simulink model "ASM_Losses"  (R2014a)
settings: Solver=ode23t  StartTime=0.0  StopTime=1/input.fs*3  MaxStep=1e-3  MinStep=1e-12  RelTol=1e-3
undefined symbols (not defined in the file or in its folder): input, motor, pwm
libraries: fl_lib x24, nesl_utility x20, elec_lib x2, simulink x2, powerlib_meascontrol x1
settings Model: Creator=sizuest  LastModifiedBy=simon
settings SolverCC: MaxConsecutiveMinStep=10
settings DataIOCC: SignalLoggingSaveFormat=ModelDataLogs
settings DebuggingCC: UnderspecifiedInitializationDetection=Classic  MaxConsecutiveZCsMsg=none  IgnoredZcDiagnostic=none  MultiTaskDSMMsg=warning  MultiTaskCondExecSysMsg=none  ParameterPrecisionLossMsg=none
settings RTWCC: IncludeERTFirstTime=on

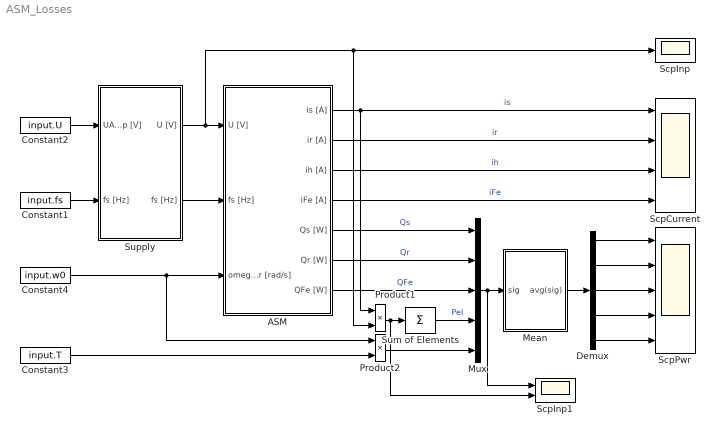
== system ASM_Losses ==
  ASM : Subsystem
  Constant1 : Constant  Value=input.fs
  Constant2 : Constant  Value=input.U
  Constant3 : Constant  Value=input.T
  Constant4 : Constant  Value=input.w0
  Demux : Demux  Outputs=5
  Mean : Subsystem
  Mux : Mux  Inputs=5
  Product1 : Product
  Product2 : Product
  ScpCurrent : Scope  NumInputPorts=4
      settings: ShowLegends=on  TimeRange=0.00432192  YMin=-100~-75~-50~-4e-06  YMax=100~75~50~4e-06  SaveName=SimOutCurrent
  ScpInp : Scope
      settings: ShowLegends=on  TimeRange=0.0101155  YMin=-400  YMax=400  SaveName=SimOutVoltage
  ScpInp1 : Scope  NumInputPorts=2
      settings: ShowLegends=on  TimeRange=0.006  YMin=-20000~-25000  YMax=65000~40000  SaveName=SimOutVoltage1
  ScpPwr : Scope  NumInputPorts=5
      settings: ShowLegends=on  TimeRange=0.00356836  YMin=0~0~-1~0~9500  YMax=700~250~1~22500~10500  SaveName=SimOutData
  Sum of Elements : Sum  Inputs=+
  Supply : Subsystem
  wires:
  ASM/6(Qr [W]) -> Mux/2  "Qr"
  ASM/5(Qs [W]) -> Mux/1  "Qs"
  Constant1/1 -> Supply/2(fs [Hz])
  Constant4/1 -> Product2/1, ASM/3(omegar [rad/s])
  Sum of Elements/1 -> Mux/4  "Pel"
  ASM/1(is [A]) -> ScpCurrent/1, Product1/1  "is"
  ASM/2(ir [A]) -> ScpCurrent/2  "ir"
  ASM/3(ih [A]) -> ScpCurrent/3  "ih"
  Supply/2("fs [Hz] ") -> ASM/2(fs [Hz])
  ASM/7(QFe [W]) -> Mux/3  "QFe"
  ASM/4(iFe [A]) -> ScpCurrent/4  "iFe"
  Supply/1(U [V]) -> Product1/2, ScpInp/1, ASM/1(U [V])
  Constant2/1 -> Supply/1(UAmp [V])
  Product1/1 -> ScpInp1/2, Sum of Elements/1
  Mux/1 -> ScpInp1/1, Mean/1(sig)
  Mean/1(avg(sig)) -> Demux/1
  Demux/3 -> ScpPwr/3
  Demux/2 -> ScpPwr/2
  Demux/1 -> ScpPwr/1
  Demux/4 -> ScpPwr/4
  Demux/5 -> ScpPwr/5
  Product2/1 -> Mux/5
  Constant3/1 -> Product2/2

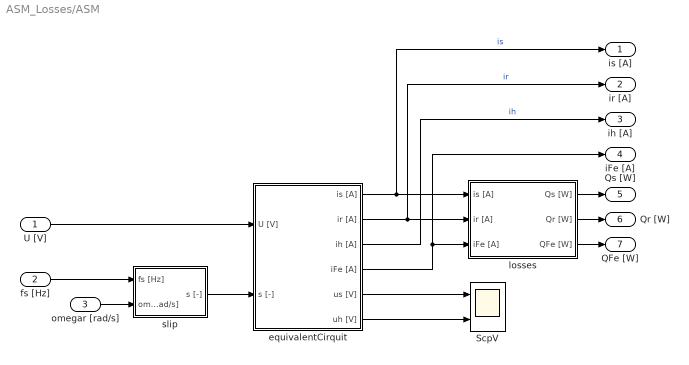
== system ASM_Losses/ASM ==
  U [V] : Inport
  fs [Hz] : Inport  Port=2
  omegar [rad/s] : Inport  Port=3
  ScpV : Scope  NumInputPorts=2
      settings: ShowLegends=on  TimeRange=0.04  YMin=-800~-550  YMax=800~550  SaveName=SimOutCurrent2
  equivalentCirquit : Subsystem
  losses : Subsystem
  slip : Subsystem
  is [A] : Outport
  ir [A] : Outport  Port=2
  ih [A] : Outport  Port=3
  iFe [A] : Outport  Port=4
  Qs [W] : Outport  Port=5
  Qr [W] : Outport  Port=6
  QFe [W] : Outport  Port=7
  wires:
  losses/2("Qr [W] ") -> Qr [W]/1
  losses/1(Qs [W]) -> Qs [W]/1
  equivalentCirquit/3(ih [A]) -> ih [A]/1  "ih"
  slip/1(s [-]) -> equivalentCirquit/2(s [-])
  fs [Hz]/1 -> slip/1(fs [Hz])
  U [V]/1 -> equivalentCirquit/1(U [V])
  equivalentCirquit/2(ir [A]) -> ir [A]/1, losses/2(ir [A])  "ir"
  equivalentCirquit/1(is [A]) -> is [A]/1, losses/1(is [A])  "is"
  losses/3(QFe [W]) -> QFe [W]/1
  equivalentCirquit/5(us [V]) -> ScpV/1
  equivalentCirquit/6(uh [V]) -> ScpV/2
  omegar [rad/s]/1 -> slip/2(omegar [rad/s])
  equivalentCirquit/4(iFe [A]) -> iFe [A]/1, losses/3(iFe [A])

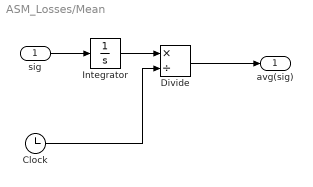
== system ASM_Losses/Mean ==
  sig : Inport
  Clock : Clock
  Divide : Product  Inputs=*/
  Integrator : Integrator
  avg(sig) : Outport
  wires:
  sig/1 -> Integrator/1
  Integrator/1 -> Divide/1
  Clock/1 -> Divide/2
  Divide/1 -> avg(sig)/1

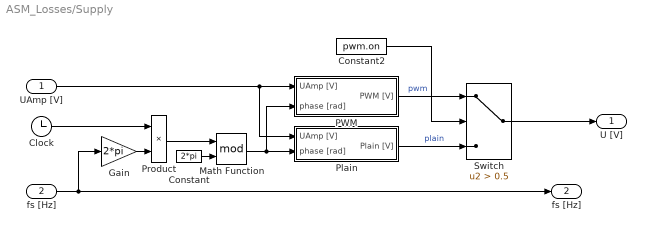
== system ASM_Losses/Supply ==
  UAmp [V] : Inport
  fs [Hz] : Inport  Port=2
  Clock : Clock
  Constant : Constant  Value=2*pi
  Constant2 : Constant  Value=pwm.on
  Gain : Gain  Gain=2*pi
  Math Function : Math  Operator=mod  SaturateOnIntegerOverflow=on
  PWM : Subsystem  mask{UAmp=pwm.Umax, fPWM=pwm.f}
      mask prompts: UAmp "Max. Amplitude [V]"; fPWM "Frequency [Hz]"
  Plain : Subsystem
  Product : Product
  Switch : Switch  Criteria=u2 > Threshold  Threshold=0.5
  U [V] : Outport
  "fs [Hz] " : Outport  Port=2
  wires:
  fs [Hz]/1 -> "fs [Hz] "/1, Gain/1
  Clock/1 -> Product/1
  Gain/1 -> Product/2
  PWM/1(PWM [V]) -> Switch/1  "pwm"
  UAmp [V]/1 -> PWM/1(UAmp [V]), Plain/1(UAmp [V])
  Math Function/1 -> Plain/2(phase [rad]), PWM/2(phase [rad])
  Plain/1(Plain [V]) -> Switch/3  "plain"
  Product/1 -> Math Function/1
  Constant/1 -> Math Function/2
  Constant2/1 -> Switch/2
  Switch/1 -> U [V]/1

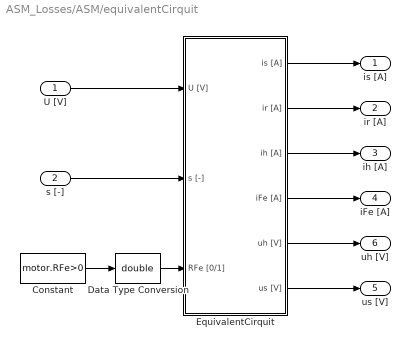
== system ASM_Losses/ASM/equivalentCirquit ==
  U [V] : Inport
  s [-] : Inport  Port=2
  Constant : Constant  Value=motor.RFe>0
  Data Type Conversion : DataTypeConversion  OutDataTypeStr=double
  EquivalentCirquit : Subsystem
  is [A] : Outport
  ir [A] : Outport  Port=2
  ih [A] : Outport  Port=3
  iFe [A] : Outport  Port=4
  us [V] : Outport  Port=5
  uh [V] : Outport  Port=6
  wires:
  U [V]/1 -> EquivalentCirquit/1(U [V])
  s [-]/1 -> EquivalentCirquit/2(s [-])
  Constant/1 -> Data Type Conversion/1
  EquivalentCirquit/1(is [A]) -> is [A]/1
  EquivalentCirquit/2(ir [A]) -> ir [A]/1
  EquivalentCirquit/3(ih [A]) -> ih [A]/1
  EquivalentCirquit/4(iFe [A]) -> iFe [A]/1
  EquivalentCirquit/5(uh [V]) -> uh [V]/1
  EquivalentCirquit/6(us [V]) -> us [V]/1
  Data Type Conversion/1 -> EquivalentCirquit/3(RFe [0/1])

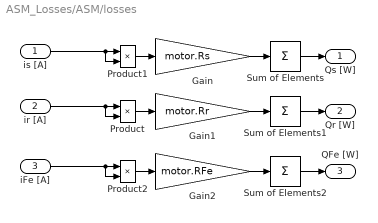
== system ASM_Losses/ASM/losses ==
  is [A] : Inport
  ir [A] : Inport  Port=2
  iFe [A] : Inport  Port=3
  Gain : Gain  Gain=motor.Rs
  Gain1 : Gain  Gain=motor.Rr
  Gain2 : Gain  Gain=motor.RFe
  Product : Product
  Product1 : Product
  Product2 : Product
  Sum of Elements : Sum  Inputs=+
  Sum of Elements1 : Sum  Inputs=+
  Sum of Elements2 : Sum  Inputs=+
  Qs [W] : Outport
  "Qr [W] " : Outport  Port=2
  QFe [W] : Outport  Port=3
  wires:
  Product1/1 -> Gain/1
  Product/1 -> Gain1/1
  Gain/1 -> Sum of Elements/1
  Gain1/1 -> Sum of Elements1/1
  Product2/1 -> Gain2/1
  Gain2/1 -> Sum of Elements2/1
  is [A]/1 -> Product1/2, Product1/1
  ir [A]/1 -> Product/2, Product/1
  iFe [A]/1 -> Product2/2, Product2/1
  Sum of Elements/1 -> Qs [W]/1
  Sum of Elements1/1 -> "Qr [W] "/1
  Sum of Elements2/1 -> QFe [W]/1

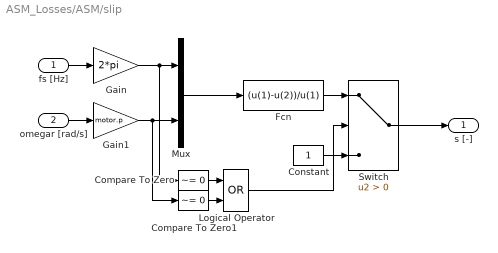
== system ASM_Losses/ASM/slip ==
  fs [Hz] : Inport
  omegar [rad/s] : Inport  Port=2
  Compare To Zero : simulink/Logic and Bit Operations/Compare To Zero  relop=~=  OutDataTypeStr=boolean
  Compare To Zero1 : simulink/Logic and Bit Operations/Compare To Zero  relop=~=  OutDataTypeStr=boolean
  Constant : Constant
  Fcn : Fcn  Expr=(u(1)-u(2))/u(1)
  Gain : Gain  Gain=2*pi
  Gain1 : Gain  Gain=motor.p
  Logical Operator : Logic  Operator=OR  AllPortsSameDT=off  OutDataTypeStr=boolean
  Mux : Mux  Inputs=2
  Switch : Switch  Criteria=u2 > Threshold
  s [-] : Outport
  wires:
  fs [Hz]/1 -> Gain/1
  omegar [rad/s]/1 -> Gain1/1
  Gain/1 -> Compare To Zero/1, Mux/1
  Gain1/1 -> Compare To Zero1/1, Mux/2
  Mux/1 -> Fcn/1
  Fcn/1 -> Switch/1
  Compare To Zero1/1 -> Logical Operator/2
  Compare To Zero/1 -> Logical Operator/1
  Constant/1 -> Switch/3
  Logical Operator/1 -> Switch/2
  Switch/1 -> s [-]/1

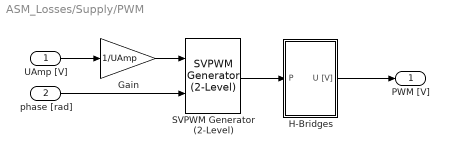
== system ASM_Losses/Supply/PWM ==
  UAmp [V] : Inport
  phase [rad] : Inport  Port=2
  Gain : Gain  Gain=1/UAmp
  H-Bridges : Subsystem
  SVPWM Generator (2-Level) : powerlib_meascontrol/Pulse & Signal Generators/SVPWM Generator (2-Level)  InputType=Magnitude-Angle (rad)  SwitchingPattern=Pattern #1  Fc=fPWM  ParUref=[10/400 0 3.7]  Ts=0
  PWM [V] : Outport
  wires:
  UAmp [V]/1 -> Gain/1
  phase [rad]/1 -> SVPWM Generator (2-Level)/2
  SVPWM Generator (2-Level)/1 -> H-Bridges/1(P)
  H-Bridges/1(U [V]) -> PWM [V]/1
  Gain/1 -> SVPWM Generator (2-Level)/1

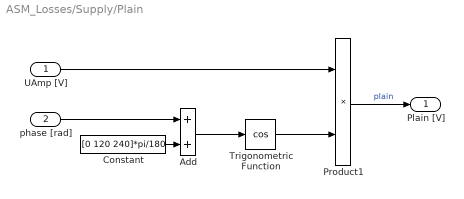
== system ASM_Losses/Supply/Plain ==
  UAmp [V] : Inport
  phase [rad] : Inport  Port=2
  Add : Sum
  Constant : Constant  Value=[0 120 240]*pi/180
  Product1 : Product
  Trigonometric Function : Trigonometry  Operator=cos
  Plain [V] : Outport
  wires:
  phase [rad]/1 -> Add/1
  UAmp [V]/1 -> Product1/1
  Product1/1 -> Plain [V]/1  "plain"
  Add/1 -> Trigonometric Function/1
  Trigonometric Function/1 -> Product1/2
  Constant/1 -> Add/2

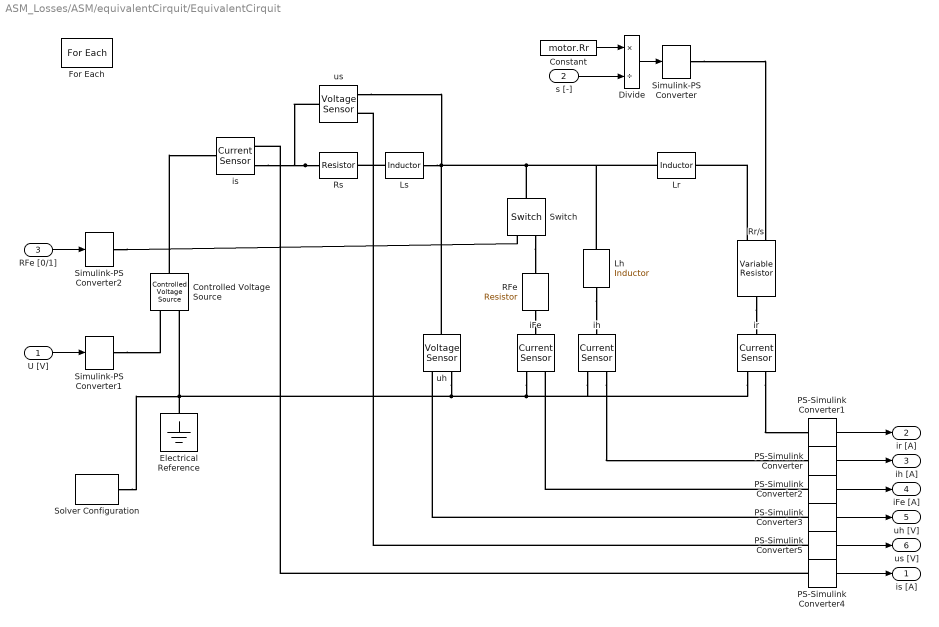
== system ASM_Losses/ASM/equivalentCirquit/EquivalentCirquit ==
  U [V] : Inport  Partition=on  PartitionDimension=1  PartitionWidth=1
  s [-] : Inport  Port=2  Partition=off
  RFe [0/1] : Inport  Port=3  Partition=off
  Constant : Constant  Value=motor.Rr
  Controlled Voltage Source : fl_lib/Electrical/Electrical Sources/Controlled Voltage Source
  Divide : Product  Inputs=*/
  Electrical Reference : fl_lib/Electrical/Electrical Elements/Electrical Reference
  For Each : ForEach  DisableCoverage=on  IndexMode=One-based
  Lh : fl_lib/Electrical/Electrical Elements/Inductor  l=motor.Lh H  r=0 Ohm  g=1e-9 1/Ohm  i_specify=off  i_priority=High  i=0 A  v_specify=off  v_priority=High  v=0 V  i_L_specify=on  i_L_priority=High  i_L=0 A
  Lr : fl_lib/Electrical/Electrical Elements/Inductor  l=motor.Lr H  r=0 Ohm  g=1e-9 1/Ohm  i_specify=off  i_priority=High  i=0 A  v_specify=off  v_priority=High  v=0 V  i_L_specify=on  i_L_priority=High  i_L=0 A
  Ls : fl_lib/Electrical/Electrical Elements/Inductor  l=motor.Ls H  r=0 Ohm  g=0 1/Ohm  i_specify=off  i_priority=High  i=0 A  v_specify=off  v_priority=High  v=0 V  i_L_specify=on  i_L_priority=High  i_L=0 A
  PS-Simulink Converter{,1..5} (6 alike) : nesl_utility/PS-Simulink Converter  PhysicalDomain=network_engine_domain  SubClassName=ps_output  LeftPortType=input  RightPortType=output  PseudoPeriodic=off  Frequencies=[]  Unit=1  AffineConversion=off
  RFe : elec_lib/Passive Devices/Resistor  R=motor.RFe Ohm  noise_mode=0  Tdevice=25 C  sample_time=0.001 s  repeatability=1  auto_seed=3499211588  user_seed=0
  Rr/s : fl_lib/Electrical/Electrical Elements/Variable Resistor  Rmin=0 Ohm  i_specify=off  i_priority=High  i=0 A  v_specify=off  v_priority=High  v=0 V
  Rs : elec_lib/Passive Devices/Resistor  R=motor.Rs Ohm  noise_mode=0  Tdevice=25 C  sample_time=0.001 s  repeatability=1  auto_seed=3890346746  user_seed=0
  Simulink-PS Converter : nesl_utility/Simulink-PS Converter  PhysicalDomain=network_engine_domain  SubClassName=ps_input  LeftPortType=input  RightPortType=output  PseudoPeriodic=off  Frequencies=[]  NoiseDistribution=none  NoiseParameters=[]  Unit=1  AffineConversion=off  InputFiltering=off  SimscapeFilterOrder=1  InputFilterTimeConstant=0.001  UdotUserProvided=1
  Simulink-PS Converter1 : nesl_utility/Simulink-PS Converter  PhysicalDomain=network_engine_domain  SubClassName=ps_input  LeftPortType=input  RightPortType=output  PseudoPeriodic=off  Frequencies=[]  NoiseDistribution=none  NoiseParameters=[]  Unit=1  AffineConversion=off  InputFiltering=off  SimscapeFilterOrder=1  InputFilterTimeConstant=0.001  UdotUserProvided=1
  Simulink-PS Converter2 : nesl_utility/Simulink-PS Converter  PhysicalDomain=network_engine_domain  SubClassName=ps_input  LeftPortType=input  RightPortType=output  PseudoPeriodic=off  Frequencies=[]  NoiseDistribution=none  NoiseParameters=[]  Unit=1  AffineConversion=off  InputFiltering=off  SimscapeFilterOrder=1  InputFilterTimeConstant=0.001  UdotUserProvided=1
  Solver Configuration : nesl_utility/Solver Configuration  PhysicalDomain=network_engine_domain  SubClassName=solver  LeftPortType=input  RightPortType=generic  Accelerate=off  Tones=[]  Harmonics=[]  SimulateNoise=off  Profile=off  UseLocalSampling=off  EnableSwitchedLinearOptims=on  FrequencyDomain=off  UseCCode=off  RelTol=0.001  AbsTol=1e-06  MinStep=1e-09  ToWorkspace=off  DoDC=off  ResidualTolerance=1e-09  UseLocalSolver=off  LocalSolverChoice=NE_BACKWARD_EULER_ADVANCER  LocalSolverSampleTime=1/500000  DoFixedCost=off  MaxNonlinIter=3  MaxModeIter=2  LinearAlgebra=Full  DelaysMemoryBudget=1024  AutomaticFiltering=on  FilteringTimeConstant=0.001
  Switch : fl_lib/Electrical/Electrical Elements/Switch  R_closed=0.001 Ohm  G_open=1e-8 1/Ohm  Threshold=0.5  i_specify=off  i_priority=High  i=0 A  v_specify=off  v_priority=High  v=0 V
  iFe : fl_lib/Electrical/Electrical Sensors/Current Sensor
  ih : fl_lib/Electrical/Electrical Sensors/Current Sensor
  ir : fl_lib/Electrical/Electrical Sensors/Current Sensor
  is : fl_lib/Electrical/Electrical Sensors/Current Sensor
  uh : fl_lib/Electrical/Electrical Sensors/Voltage Sensor
  us : fl_lib/Electrical/Electrical Sensors/Voltage Sensor
  is [A] : Outport  ConcatenationDimension=1
  ir [A] : Outport  Port=2  ConcatenationDimension=1
  ih [A] : Outport  Port=3  ConcatenationDimension=1
  iFe [A] : Outport  Port=4  ConcatenationDimension=1
  uh [V] : Outport  Port=5  ConcatenationDimension=1
  us [V] : Outport  Port=6  ConcatenationDimension=1
  wires:
  PS-Simulink Converter/1 -> ih [A]/1
  s [-]/1 -> Divide/2
  PS-Simulink Converter2/1 -> iFe [A]/1
  PS-Simulink Converter5/1 -> us [V]/1
  PS-Simulink Converter3/1 -> uh [V]/1
  U [V]/1 -> Simulink-PS Converter1/1
  Divide/1 -> Simulink-PS Converter/1
  PS-Simulink Converter1/1 -> ir [A]/1
  PS-Simulink Converter4/1 -> is [A]/1
  Constant/1 -> Divide/1
  RFe [0/1]/1 -> Simulink-PS Converter2/1
  connections:
  Lh/RConn1 -- ih/LConn1
  Rs/LConn1 -- is/RConn2 -- us/LConn1
  Solver Configuration/RConn1 -- Controlled Voltage Source/RConn2 -- Electrical Reference/LConn1 -- uh/RConn2 -- ir/RConn2 -- ih/RConn2 -- iFe/RConn2
  Rr/s/RConn1 -- ir/LConn1
  ih/RConn1 -- PS-Simulink Converter/LConn1
  RFe/RConn1 -- iFe/LConn1
  PS-Simulink Converter2/LConn1 -- iFe/RConn1
  Simulink-PS Converter/RConn1 -- Rr/s/LConn1
  Simulink-PS Converter1/RConn1 -- Controlled Voltage Source/RConn1
  Controlled Voltage Source/LConn1 -- is/LConn1
  ir/RConn1 -- PS-Simulink Converter1/LConn1
  PS-Simulink Converter5/LConn1 -- us/RConn1
  PS-Simulink Converter4/LConn1 -- is/RConn1
  Switch/LConn1 -- Lh/LConn1 -- Lr/LConn1 -- us/RConn2 -- Ls/RConn1 -- uh/LConn1
  Ls/LConn1 -- Rs/RConn1
  PS-Simulink Converter3/LConn1 -- uh/RConn1
  Rr/s/LConn2 -- Lr/RConn1
  Switch/RConn2 -- RFe/LConn1
  Simulink-PS Converter2/RConn1 -- Switch/RConn1

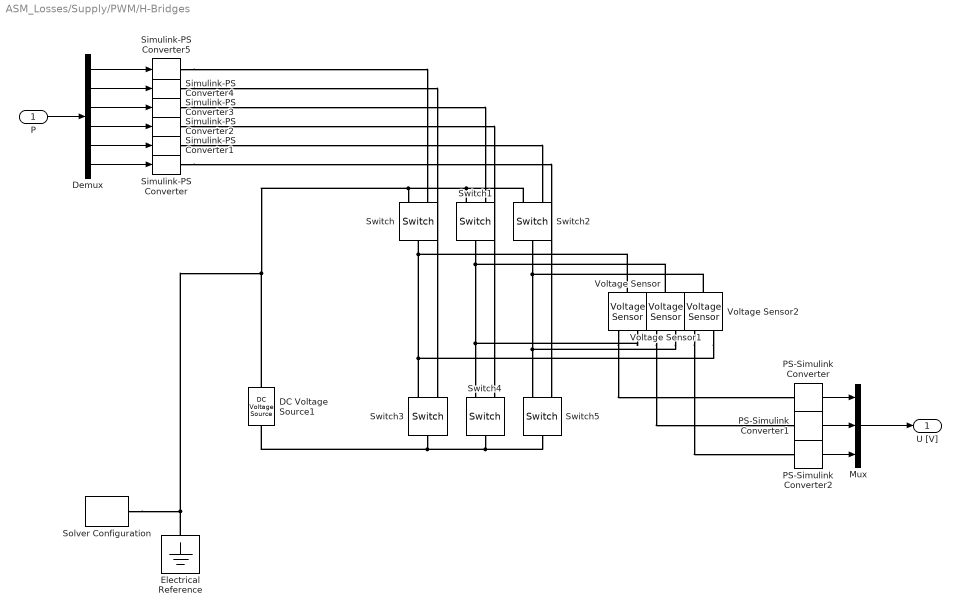
== system ASM_Losses/Supply/PWM/H-Bridges ==
  P : Inport
  DC Voltage Source1 : fl_lib/Electrical/Electrical Sources/DC Voltage Source  v0=UAmp V
  Demux : Demux  Outputs=6
  Electrical Reference : fl_lib/Electrical/Electrical Elements/Electrical Reference
  Mux : Mux  Inputs=3
  PS-Simulink Converter : nesl_utility/PS-Simulink Converter  PhysicalDomain=network_engine_domain  SubClassName=ps_output  LeftPortType=input  RightPortType=output  PseudoPeriodic=off  Frequencies=[]  Unit=1  AffineConversion=off
  PS-Simulink Converter1 : nesl_utility/PS-Simulink Converter  PhysicalDomain=network_engine_domain  SubClassName=ps_output  LeftPortType=input  RightPortType=output  PseudoPeriodic=off  Frequencies=[]  Unit=1  AffineConversion=off
  PS-Simulink Converter2 : nesl_utility/PS-Simulink Converter  PhysicalDomain=network_engine_domain  SubClassName=ps_output  LeftPortType=input  RightPortType=output  PseudoPeriodic=off  Frequencies=[]  Unit=1  AffineConversion=off
  Simulink-PS Converter{,1..5} (6 alike) : nesl_utility/Simulink-PS Converter  PhysicalDomain=network_engine_domain  SubClassName=ps_input  LeftPortType=input  RightPortType=output  PseudoPeriodic=off  Frequencies=[]  NoiseDistribution=none  NoiseParameters=[]  Unit=1  AffineConversion=off  InputFiltering=off  SimscapeFilterOrder=1  InputFilterTimeConstant=0.001  UdotUserProvided=1
  Solver Configuration : nesl_utility/Solver Configuration  PhysicalDomain=network_engine_domain  SubClassName=solver  LeftPortType=input  RightPortType=generic  Accelerate=off  Tones=[]  Harmonics=[]  SimulateNoise=off  Profile=off  UseLocalSampling=off  EnableSwitchedLinearOptims=on  FrequencyDomain=off  UseCCode=off  RelTol=0.001  AbsTol=1e-06  MinStep=1e-09  ToWorkspace=off  DoDC=off  ResidualTolerance=1e-09  UseLocalSolver=off  LocalSolverChoice=NE_BACKWARD_EULER_ADVANCER  LocalSolverSampleTime=0.001  DoFixedCost=off  MaxNonlinIter=3  MaxModeIter=2  LinearAlgebra=Sparse  DelaysMemoryBudget=1024  AutomaticFiltering=on  FilteringTimeConstant=0.001
  Switch{,1..5} (6 alike) : fl_lib/Electrical/Electrical Elements/Switch  R_closed=0.01 Ohm  G_open=1e-8 1/Ohm  Threshold=0  i_specify=off  i_priority=High  i=0 A  v_specify=off  v_priority=High  v=0 V
  Voltage Sensor : fl_lib/Electrical/Electrical Sensors/Voltage Sensor
  Voltage Sensor1 : fl_lib/Electrical/Electrical Sensors/Voltage Sensor
  Voltage Sensor2 : fl_lib/Electrical/Electrical Sensors/Voltage Sensor
  U [V] : Outport
  wires:
  PS-Simulink Converter2/1 -> Mux/3
  PS-Simulink Converter1/1 -> Mux/2
  PS-Simulink Converter/1 -> Mux/1
  Mux/1 -> U [V]/1
  P/1 -> Demux/1
  Demux/1 -> Simulink-PS Converter5/1
  Demux/2 -> Simulink-PS Converter4/1
  Demux/3 -> Simulink-PS Converter3/1
  Demux/4 -> Simulink-PS Converter2/1
  Demux/5 -> Simulink-PS Converter1/1
  Demux/6 -> Simulink-PS Converter/1
  connections:
  Switch/RConn2 -- Solver Configuration/RConn1 -- Electrical Reference/LConn1 -- DC Voltage Source1/LConn1 -- Switch1/RConn2 -- Switch2/RConn2
  Switch/LConn1 -- Voltage Sensor2/RConn2 -- Switch3/RConn2 -- Voltage Sensor/LConn1
  Switch1/LConn1 -- Voltage Sensor1/LConn1 -- Voltage Sensor/RConn2 -- Switch4/RConn2
  Switch2/LConn1 -- Voltage Sensor2/LConn1 -- Voltage Sensor1/RConn2 -- Switch5/RConn2
  DC Voltage Source1/RConn1 -- Switch3/LConn1 -- Switch5/LConn1 -- Switch4/LConn1
  Simulink-PS Converter5/RConn1 -- Switch/RConn1
  Simulink-PS Converter4/RConn1 -- Switch3/RConn1
  Simulink-PS Converter3/RConn1 -- Switch1/RConn1
  Simulink-PS Converter2/RConn1 -- Switch4/RConn1
  Simulink-PS Converter1/RConn1 -- Switch2/RConn1
  Simulink-PS Converter/RConn1 -- Switch5/RConn1
  Voltage Sensor/RConn1 -- PS-Simulink Converter/LConn1
  Voltage Sensor1/RConn1 -- PS-Simulink Converter1/LConn1
  Voltage Sensor2/RConn1 -- PS-Simulink Converter2/LConn1
